simulink model "buck_fo_lqi_fixed_reference_v6_1_46V_R2022a"  (R2022a)
settings: Solver=ode23tb  StartTime=0.0  StopTime=Tsim  MaxStep=2e-7  RelTol=1e-6  AbsTol=1e-8
InitFcn:
  | f=get_param(bdroot,'FileName');addpath(fullfile(fileparts(fileparts(f)),'matlab'));clear f
model workspace (MAT data in the model file):
  C = 0.0001
  COMPARATOR_MISSION_SCOPE = 'Wide-range 1-46 V mission. The 1-V setpoint sits 3 % from the CCM/DCM boundary at the nominal 10 ohm load, and the 24 -> 1 V step forces about 3.2 ms of discontinuous operation.'
  COMPARATOR_REVISION = 'v6-wide-range-fixed-reference-common-layer-r1'
  COMPARATOR_SYNTHESIS_RULE = 'Buck adaptation of published FO-LQI architecture; classical Bryson LQI gain, fixed fractional order 0.781'
  CONTROLLER_ARCHITECTURE = 'FO_LQI_fixed_reference'
  CONTROLLER_CODE = 6
  CTRL_PARAM_VECTOR = [6 0 0 0.0329680242646 0.0102858294154 -90.2361993135 0 1e-05 9424.77796077 0.02 0.98 10 0.1 0.02 0.05 0.42 32401 0.000106103295395 0.48 48000 0.05 0.511044924299 0.781 0 0 0 0 0 0 0 0 0 0 24]
  CURRENT_CONVENTION = 'iC downward; iL=i_out_branch+iC; i_out_branch=iR+iPert'
  Cs = inf
  DEVICE_MODEL_SCOPE = 'Static affine conduction model from the manufacturer loss law. Reverse leakage, junction capacitance, package parasitics, thermal feedback and commutation transients require a separate device model.'
  ENERGY_ACCOUNTING = 'Pin=Vin*iin; useful load=vout^2/R+vout*ipert; losses=rL*iL^2+rC*iC^2+vSW*iSW+vD*iD+vSW^2/Rs'
  ENERGY_AUDIT_REVISION = '2026-09-12-IRF540N-STPST10H100-static-conduction-r1'
  FREEWHEEL_DIODE_DATASHEET = 'https://www.st.com/resource/en/datasheet/stpst10h100.pdf'
  FREEWHEEL_DIODE_PART = 'STPST10H100SF'
  HIGH_SIDE_DEVICE_TECHNOLOGY = 'MOSFET'
  Iload_amp = 0.5
  Iload_ts = [0  0; 0.053999999  0; 0.054  0.5; 0.089999999  0.5; 0.09  0; 0.324  0]
  Kb = 9424.77796077
  Kd = 3.50371189288e-06
  Ki = 98.3455091559
  Kp = 0.0156901027664
  L = 0.0001
  MODEL_AUDIT_REVISION = '2026-09-06-current-sign-r1'
  Nf = 200000
  OPTIMIZED_BY_CMO_FRAMEWORK = 0
  R = 10
  Ron = 0.05
  Rs = 100000
  SWITCH_PART = 'IRF540N/IRF540NPbF'
  Te = 1e-05
  Tsim = 0.324
  Tt = 0.000115
  VIN_POLICY = 'Vin=48 V constant in the main study'
  Vf = 0.42
  Vin = 48
  Vin_lvl = [48 48 48]
  Vin_nom = 48
  Vin_ts = [0  48; 0.107999999  48; 0.108  48; 0.215999999  48; 0.216  48; 0.324  48]
  Vref_lvl = [24 1 46]
  Vref_ts = [0  24; 0.107999999  24; 0.108  1; 0.215999999  1; 0.216  46; 0.324  46]
  b = 1
  c = 0
  d_max = 0.98
  d_min = 0.02
  fs = 50000
  rC = 0.05
  rL = 0.1
  rd = 0.02
  t_sw = [0.108 0.216]
libraries: spsParallelRLCBranchLib x4, spsCurrentMeasurementLib x3, spsVoltageMeasurementLib x2, spsControlledVoltageSourceLib x1, spsDiodeLib x1, spsPWMGeneratorDCDCLib x1, spsMosfetLib x1, spsSeriesRLCBranchLib x1, spsControlledCurrentSourceLib x1, spspowerguiLib x1
Description:
  | Buck non ideal corrige selon la Table 1. Vin=48 V constant. PIDF 2-DOF: r=Vref, y=Vo, b=c=0. Saturation duty total, tracking anti-windup, journal q(t), reconstruction iL=iR+iC, source de perturbation de charge et solveur ode23tb.
  | Energy audit r2: direct IGBT/diode voltage-current logs; active controller renamed from misleading LQI Command to PIDF 2DOF Command. Vin remains constant at 48 V.
  | Revised device layer: high-side IRF540N MOSFET topology and STPST10H100SF freewheel diode. Static diode parameters are taken from the ST conduction-loss equation; thermal and detailed commutation dynamics are not represented.
  | Wide-range fixed reference comparator: FO_LQI_fixed_reference. Parameters are frozen by the declared synthesis rule and are not optimized by the proposed methodology.
settings Model: Creator=adolphejunior  LastModifiedBy=adolphejunior

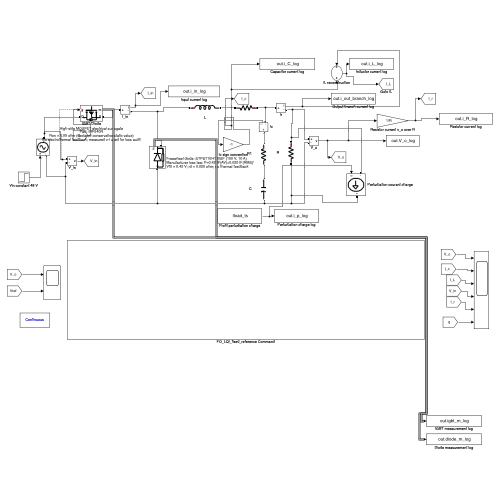
[thumbnail: Simulink's stored preview of the top-level diagram]
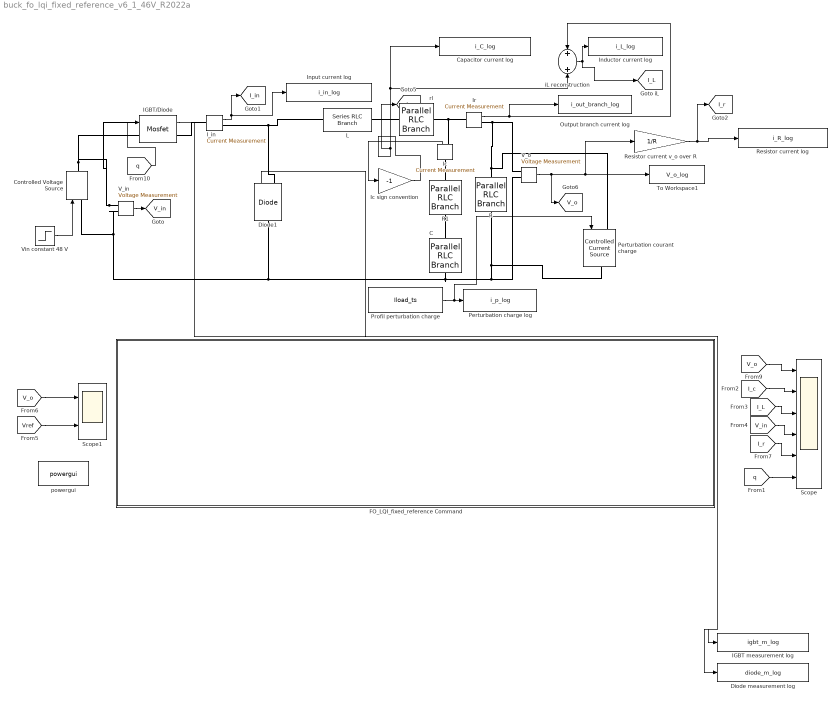
== system buck_fo_lqi_fixed_reference_v6_1_46V_R2022a ==
  C : spsParallelRLCBranchLib/Parallel RLC Branch  LConnTagsString=a  RConnTagsString=__new0  BranchType=C  Resistance=1  Inductance=1e-3  SetiL0=off  InitialCurrent=0  Capacitance=100e-6  Setx0=on  InitialVoltage=12  Measurements=None
  Capacitor current log : ToWorkspace  VariableName=i_C_log  SaveFormat=Timeseries  SampleTime=-1
  Controlled Voltage Source : spsControlledVoltageSourceLib/Controlled Voltage Source  Initialize=on  Source_Type=DC  Amplitude=0  Phase=0  Frequency=0  Measurements=None
  Diode measurement log : ToWorkspace  VariableName=diode_m_log  SaveFormat=Timeseries  SampleTime=-1
  Diode1 : spsDiodeLib/Diode  Ron=rd  Lon=0  Vf=Vf  IC=0  UseSnubber=0  Rs=Rs  Cs=Cs  Measurements=on
      settings: AttributesFormatString=|
      | Freewheel diode: STPST10H100SF (100 V, 10 A)
      | Manufacturer loss law: P=0.42 IF(AV)+0.020 IF(RMS)^2
      | Vf0 = 0.42 V; rd = 0.020 ohm; no thermal feedback
  FO_LQI_fixed_reference Command : Subsystem
  IGBT measurement log : ToWorkspace  VariableName=igbt_m_log  SaveFormat=Timeseries  SampleTime=-1
  IGBT/Diode : spsMosfetLib/Mosfet  Ron=Ron  Lon=0  Rd=0.01  Vfd=0  IC=0  Rs=Rs  Cs=Cs  Measurements=on
      settings: AttributesFormatString=|
      | High-side MOSFET electrical surrogate
      | Part: IRF540N
      | Ron = 0.05 ohm (declared conservative static value)
      | No electrothermal feedback; measured v-i used for loss audit
  I_in : spsCurrentMeasurementLib/Current Measurement  PhasorSimulation=off  OutputType=Complex  PSBequivalent=0
  Ic : spsCurrentMeasurementLib/Current Measurement  PhasorSimulation=off  OutputType=Complex  PSBequivalent=0
  Ic sign convention : Gain  Gain=-1
  Inductor current log : ToWorkspace  VariableName=i_L_log  SaveFormat=Timeseries  SampleTime=-1
  Input current log : ToWorkspace  VariableName=i_in_log  SaveFormat=Timeseries  SampleTime=-1
  Ir : spsCurrentMeasurementLib/Current Measurement  PhasorSimulation=off  OutputType=Complex  PSBequivalent=0
  L : spsSeriesRLCBranchLib/Series RLC Branch  LConnTagsString=__new0  RConnTagsString=__new0  BranchType=L  Resistance=1  Inductance=100e-6  SetiL0=on  InitialCurrent=1.2  Capacitance=1e-6  Setx0=off  InitialVoltage=0  Measurements=None
  Output branch current log : ToWorkspace  VariableName=i_out_branch_log  SaveFormat=Timeseries  SampleTime=-1
  Perturbation charge log : ToWorkspace  VariableName=i_p_log  SaveFormat=Timeseries  SampleTime=-1
  Perturbation courant charge : spsControlledCurrentSourceLib/Controlled Current Source  Initialize=on  Source_Type=AC  Amplitude=0  Phase=0  Frequency=0  Measurements=None
  Profil perturbation charge : FromWorkspace  VariableName=Iload_ts  Interpolate=off  OutputAfterFinalValue=Holding final value
  R : spsParallelRLCBranchLib/Parallel RLC Branch  LConnTagsString=a  RConnTagsString=__new0  BranchType=R  Resistance=10  Inductance=1e-3  SetiL0=off  InitialCurrent=0  Capacitance=1e-6  Setx0=off  InitialVoltage=0  Measurements=None
  R1 : spsParallelRLCBranchLib/Parallel RLC Branch  LConnTagsString=a  RConnTagsString=__new0  BranchType=R  Resistance=0.05  Inductance=1e-3  SetiL0=off  InitialCurrent=0  Capacitance=1e-6  Setx0=off  InitialVoltage=0  Measurements=None
  Resistor current log : ToWorkspace  VariableName=i_R_log  SaveFormat=Timeseries  SampleTime=-1
  Resistor current v_o over R : Gain  Gain=1/R
  Scope : Scope  NumInputPorts=6
  Scope1 : Scope  NumInputPorts=2
  To Workspace1 : ToWorkspace  VariableName=V_o_log  SaveFormat=Timeseries  SampleTime=-1
  V_in : spsVoltageMeasurementLib/Voltage Measurement  PhasorSimulation=off  OutputType=Complex  PSBequivalent=0
  V_o : spsVoltageMeasurementLib/Voltage Measurement  PhasorSimulation=off  OutputType=Complex  PSBequivalent=0
  Vin constant 48 V : Step  Before=48  After=48  SampleTime=0
  iL reconstruction : Sum
  powergui : spspowerguiLib/powergui  Priority=1  SimulationMode=Continuous  SampleTime=1e-6  frequency=60  Iterations=50  frequencyindice=0  Pbase=100e6  ErrMax=1e-4  UnitsV=kV  UnitsW=MW  buscounter=0  FunctionMessages=off  echomessages=off  EnableUseOfTLC=off  CurrentSourceSwitches=off  DisableSnubberDevices=off  DisableRonSwitches=off  DisableVfSwitches=off  DisplayEquations=off  AutomaticDiscreteSolvers=off  SolverType=Tustin/Backward Euler (TBE)  Interpol=off  ExternalGateDelay=off  methode=off  Ts=100  x0status=blocks  SPID=on  SwTol=0  HookPort=off  NonlinearTolerance=1e-4  nMaxIteration=100  ContinueOnMaxIteration=off  RestoreLinks=warning  ResistiveCurrentMeasurement=off  Frange=[0:2:500]  Ylog=off  Xlog=on  ShowGrid=off  save=off  variable=ZData  structure=0  ZoomFFT=off  StartTime=0.0  cycles=1  DisplayStyle=1  fundamental=60  FreqAxis=off  MaxFrequency=1000  frequencyindicesteady=1  RmsSteady=1  display=off
  rl : spsParallelRLCBranchLib/Parallel RLC Branch  LConnTagsString=a  RConnTagsString=__new0  BranchType=R  Resistance=0.1  Inductance=1e-3  SetiL0=off  InitialCurrent=0  Capacitance=1e-6  Setx0=off  InitialVoltage=0  Measurements=None
  tag scope: I_L=global, I_c=global, I_in=global, I_r=global, V_in=global, V_o=global
  wires:
  Ir/1 -> Output branch current log/1, iL reconstruction/1
  [V_o] -> Scope1/1
  [Vref] -> Scope1/2
  I_in/1 -> [I_in], Input current log/1
  [I_r] -> Scope/5
  [I_L] -> Scope/3
  V_in/1 -> [V_in]
  V_o/1 -> Resistor current v_o over R/1, To Workspace1/1, [V_o]
  [q] -> Scope/6
  [I_c] -> Scope/2
  [V_in] -> Scope/4
  iL reconstruction/1 -> [I_L], Inductor current log/1
  Vin constant 48 V/1 -> Controlled Voltage Source/1
  Profil perturbation charge/1 -> Perturbation courant charge/1, Perturbation charge log/1
  Ic/1 -> Ic sign convention/1
  Ic sign convention/1 -> Capacitor current log/1, iL reconstruction/2, [I_c]
  Resistor current v_o over R/1 -> Resistor current log/1, [I_r]
  [V_o] -> Scope/1
  Diode1/1 -> Diode measurement log/1
  [q] -> IGBT/Diode/1
  IGBT/Diode/1 -> IGBT measurement log/1
  connections:
  Ir/RConn1 -- V_o/LConn1 -- R/LConn1 -- Perturbation courant charge/LConn1
  Ic/RConn1 -- Ir/LConn1 -- rl/LConn1
  Controlled Voltage Source/LConn1 -- Diode1/LConn1 -- V_o/LConn2 -- R/RConn1 -- Perturbation courant charge/RConn1 -- C/RConn1 -- V_in/LConn2
  rl/RConn1 -- L/RConn1
  R1/LConn1 -- Ic/LConn1
  R1/RConn1 -- C/LConn1
  L/LConn1 -- Diode1/RConn1 -- I_in/RConn1
  V_in/LConn1 -- Controlled Voltage Source/RConn1 -- IGBT/Diode/LConn1
  IGBT/Diode/RConn1 -- I_in/LConn1

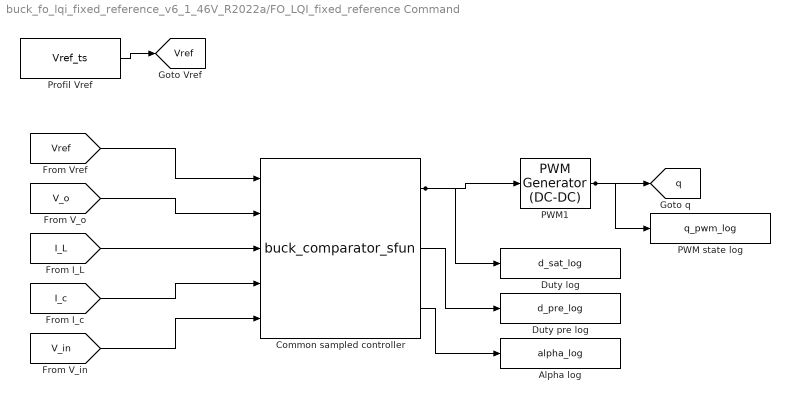
== system buck_fo_lqi_fixed_reference_v6_1_46V_R2022a/FO_LQI_fixed_reference Command ==
  Alpha log : ToWorkspace  VariableName=alpha_log  SaveFormat=Timeseries  SampleTime=-1
  Common sampled controller : M-S-Function  FunctionName=buck_comparator_sfun  Parameters=CTRL_PARAM_VECTOR
  Duty log : ToWorkspace  VariableName=d_sat_log  SaveFormat=Timeseries  SampleTime=-1
  Duty pre log : ToWorkspace  VariableName=d_pre_log  SaveFormat=Timeseries  SampleTime=-1
  PWM state log : ToWorkspace  VariableName=q_pwm_log  SaveFormat=Timeseries  SampleTime=-1
  PWM1 : spsPWMGeneratorDCDCLib/PWM Generator (DC-DC)  Fsw=50000  Ts=0
  Profil Vref : FromWorkspace  VariableName=Vref_ts  Interpolate=off  OutputAfterFinalValue=Holding final value
  tag scope: Vref=global, q=global
  wires:
  Profil Vref/1 -> [Vref]
  [Vref] -> Common sampled controller/1
  [V_o] -> Common sampled controller/2
  [I_L] -> Common sampled controller/3
  [I_c] -> Common sampled controller/4
  [V_in] -> Common sampled controller/5
  Common sampled controller/1 -> PWM1/1, Duty log/1
  Common sampled controller/2 -> Duty pre log/1
  Common sampled controller/3 -> Alpha log/1
  PWM1/1 -> [q], PWM state log/1
